simulink model "pred_prey"  (R2023a)
settings: Solver=VariableStepAuto  StartTime=0.0  StopTime=500  RelTol=1e-3
undefined symbols (not defined in the file): a, b, c, d, r
settings Model: Creator=brian  LastModifiedBy=brian

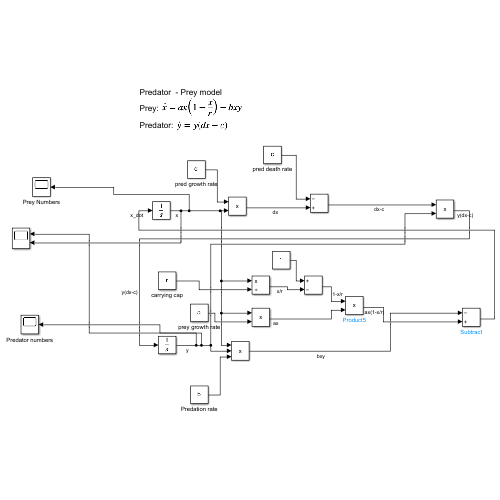
[thumbnail: Simulink's stored preview of the top-level diagram]
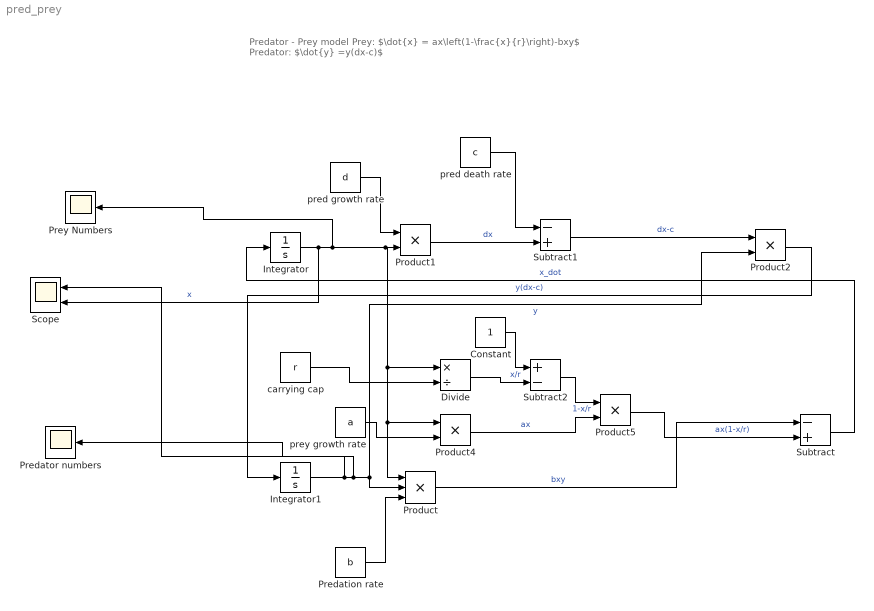
== system pred_prey ==
  note: Predator - Prey model
      | Prey: $\dot{x} = ax\left(1-\frac{x}{r}\right)-bxy$
      | Predator: $\dot{y} =y(dx-c)$
  Constant : Constant
  Divide : Product  Inputs=*/
  Integrator : Integrator  InitialCondition=19000
  Integrator1 : Integrator  InitialCondition=25
  Predation rate : Constant  Value=b
  Predator numbers : Scope
  Prey Numbers : Scope
  Product : Product  Inputs=3
  Product{1..2,4..5} (4 alike) : Product
  Scope : Scope  NumInputPorts=2
  Subtract : Sum  Inputs=-+
  Subtract1 : Sum  Inputs=-+
  Subtract2 : Sum  Inputs=+-
  carrying cap : Constant  Value=r
  pred death rate : Constant  Value=c
  pred growth rate : Constant  Value=d
  prey growth rate : Constant  Value=a
  wires:
  Integrator1/1 -> Predator numbers/1, Scope/1, Product/2, Product2/2  "y"
  Integrator/1 -> Scope/2, Prey Numbers/1, Product4/1, Product/1, Divide/1, Product1/2  "x"
  pred growth rate/1 -> Product1/1
  Predation rate/1 -> Product/3
  Product/1 -> Subtract/1  "bxy"
  Product1/1 -> Subtract1/2  "dx"
  pred death rate/1 -> Subtract1/1
  Subtract1/1 -> Product2/1  "dx-c"
  Product2/1 -> Integrator1/1  "y(dx-c)"
  Subtract/1 -> Integrator/1  "x_dot"
  prey growth rate/1 -> Product4/2
  Product4/1 -> Product5/2  "ax"
  carrying cap/1 -> Divide/2
  Divide/1 -> Subtract2/2  "x/r"
  Constant/1 -> Subtract2/1
  Subtract2/1 -> Product5/1  "1-x/r"
  Product5/1 -> Subtract/2  "ax(1-x/r)"
